simulink model "Autopilot"  (R2024a)
settings: Solver=ode4  StartTime=0.0  StopTime=1800  FixedStep=0.01  RelTol=1e-3
values from neighbouring files (symbols this model uses):
  A_lateral = [Yv, Yp+wo, Yr-u_0, g*cos(theta_0), 0 ... (first row only)    [main.m]
  A_longitudinal = [Xu, Xw,-w_0, -g*cos(theta_0) ... (first row only)    [main.m]
  B_lateral = [Yda, Ydr ... (first row only)    [main.m]
  B_longitudinal = [Xde, Xth ... (first row only)    [main.m]
  C_lateral = eye(5)    [main.m]
  C_longitudinal = eye(4)    [main.m]
  Control_Matrix = [0 Xde Xth 0 ... (first row only)    [main.m]
  D2R = pi/180    (= 0.0174532925199)    [main.m]
  D_lateral = zeros(5, 2)    [main.m]
  D_longitudinal = zeros(4, 2)    [main.m]
  g = aircraft_data(52)    [main.m]
  G = 1/(1-Ixz^2/(Ixx*Izz))    [LateralFunc.m]
  Ixx = aircraft_data(53)    [main.m]
  Iyy = aircraft_data(54)    [main.m]
  Izz = aircraft_data(55)    [main.m]
  m = aircraft_data(51)    [main.m]
  M_0 = [0;0;0]    [main.m]
  mg0 = m * g * [sin(s0(8)); -cos(s0(8)) * sin(s0(7)); -cos(s0(8)) * cos(s0(7))]    [main.m]
  p_0 = s0(4)    [main.m]
  phi_0 = s0(7)    [F_M_Calculation.m]    (also in main.m)
  psi_0 = s0(9)    [F_M_Calculation.m]    (also in main.m)
  q_0 = s0(5)    [main.m]
  R2D = 180/pi    (= 57.2957795131)    [main.m]
  r_0 = s0(6)    [main.m]
  s0 = aircraft_data(4:15)    [main.m]
  State_Matrix = [ Xu  0   Xw  0   0   0   0 ... (first row only)    [main.m]
  theta_0 = s0(8)    [F_M_Calculation.m]    (also in main.m)
  u_0 = s0(1)    [main.m]
  v_0 = s0(2)    [main.m]
  w_0 = s0(3)    [main.m]
  z_0 = s0(12)    [main.m]
undefined symbols (not defined in the file or in its folder): Earth, Receive, Send, so_struct, WGS84
libraries: cstblocks x20, simulink x3, aerolibfltsims x2, aerolibasang x2, aerolibtransform2 x1, SignalEditorBlockLib x1, shared6dof x1, dspsigops x1
settings Model: Creator=Abdelateef  LastModifiedBy=Abdelateef

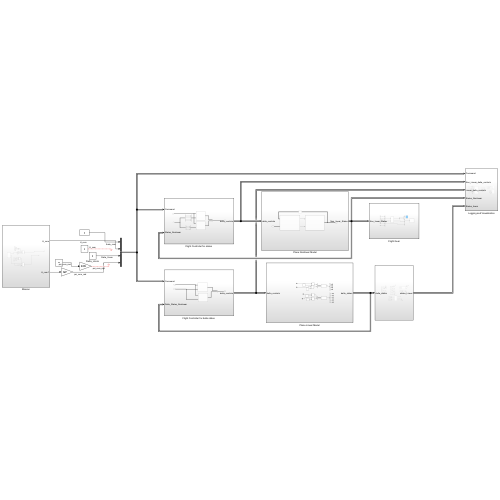
[thumbnail: Simulink's stored preview of the top-level diagram]
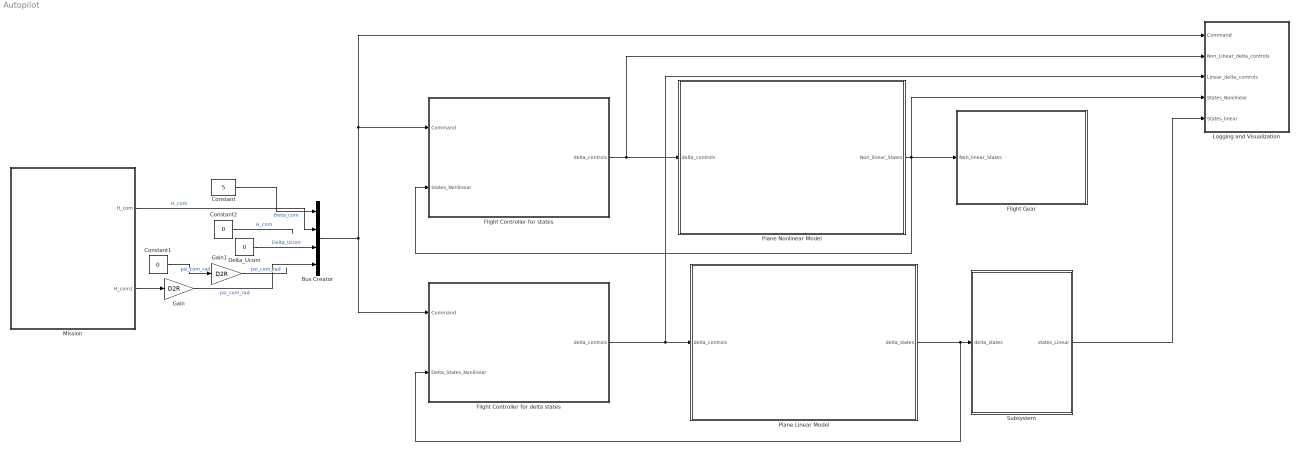
== system Autopilot ==
  Bus Creator : BusCreator  Inputs=4
  Constant : Constant  Value=5
  Constant1 : Constant  Value=0
  Constant2 : Constant  Value=0
  Delta_Ucom : Constant  Value=0
  "Flight Controller for delta states " : Subsystem
  "Flight Controller for states " : Subsystem
  Flight Gear : Subsystem
  Gain : Gain  Gain=D2R
  Gain1 : Gain  Gain=D2R
  Logging and Visualization : Subsystem
  Mission : Subsystem
  Plane Linear Model : Subsystem
  Plane Nonlinear Model : Subsystem
  Subsystem : Subsystem
  wires:
  "Flight Controller for states "/1(delta_controls) -> Logging and Visualization/2(Non_Linear_delta_controls), Plane Nonlinear Model/1(delta_controls)
  Plane Nonlinear Model/1(Non_linear_States) -> "Flight Controller for states "/2(States_Nonlinear), Flight Gear/1(Non_linear_States), Logging and Visualization/4(States_Nonlinear)
  Plane Linear Model/1(delta_states) -> "Flight Controller for delta states "/2(Delta_States_Nonlinear), Subsystem/1(delta_states)
  Bus Creator/1 -> Logging and Visualization/1(Command), "Flight Controller for states "/1(Command), "Flight Controller for delta states "/1(Command)
  "Flight Controller for delta states "/1(delta_controls) -> Logging and Visualization/3(Linear_delta_controls), Plane Linear Model/1(delta_controls)
  Gain/1 -> Bus Creator/4  "psi_com_rad"
  Delta_Ucom/1 -> Bus Creator/3  "Delta_Ucom"
  Subsystem/1(states_Linear) -> Logging and Visualization/5(States_linear)
  Constant1/1 -> Gain1/1  "psi_com_rad"
  Constant/1 -> Bus Creator/1  "theta_com"
  Gain1/1 -> ?  "psi_com_rad"
  Constant2/1 -> ?  "H_com"
  Mission/1(H_com) -> Bus Creator/2  "H_com"
  Mission/2(H_com1) -> Gain/1

== system Autopilot/Flight Controller for delta states  ==
  Command : Inport
  Delta_States_Nonlinear : Inport  Port=2
  Bus Creator : BusCreator  Inputs=2
  Lateral Controller : Subsystem
  Longitudinal Controller : Subsystem
  delta_controls : Outport
  wires:
  Lateral Controller/1(Latr_control_actions) -> Bus Creator/2  "Latr_control_actions"
  Longitudinal Controller/1(long_control_actions) -> Bus Creator/1  "long_control_actions"
  Bus Creator/1 -> delta_controls/1
  Command/1 -> Lateral Controller/1(Command), Longitudinal Controller/1(Command)
  Delta_States_Nonlinear/1 -> Lateral Controller/2(delta_states), Longitudinal Controller/2(delta_states)

== system Autopilot/Flight Controller for states  ==
  Command : Inport
  States_Nonlinear : Inport  Port=2
  Bus Creator : BusCreator  Inputs=5
  Bus Creator1 : BusCreator  Inputs=3
  Bus Creator2 : BusCreator  Inputs=2
  Bus Selector : BusSelector  OutputSignals=u,w,q,theta,H
  Bus Selector1 : BusSelector  OutputSignals=phi,psi,r
  Lateral Controller : Subsystem
  Longitudinal Controller : Subsystem
  delta_controls : Outport
  wires:
  Lateral Controller/1(Latr_control_actions) -> Bus Creator2/2  "Latr_control_actions"
  Longitudinal Controller/1(long_control_actions) -> Bus Creator2/1  "long_control_actions"
  Bus Creator2/1 -> delta_controls/1
  Command/1 -> Lateral Controller/1(Command), Longitudinal Controller/1(Command)
  States_Nonlinear/1 -> Bus Selector/1, Bus Selector1/1
  Bus Selector/1 -> Bus Creator/1  "<u>"
  Bus Selector/2 -> Bus Creator/2  "<w>"
  Bus Selector/3 -> Bus Creator/3  "<q>"
  Bus Selector/4 -> Bus Creator/4  "<theta>"
  Bus Selector/5 -> Bus Creator/5  "<H>"
  Bus Creator/1 -> Longitudinal Controller/2(States_long)
  Bus Selector1/3 -> Bus Creator1/3  "<r>"
  Bus Selector1/2 -> Bus Creator1/2  "<psi>"
  Bus Selector1/1 -> Bus Creator1/1  "<phi>"
  Bus Creator1/1 -> Lateral Controller/2(States_later)

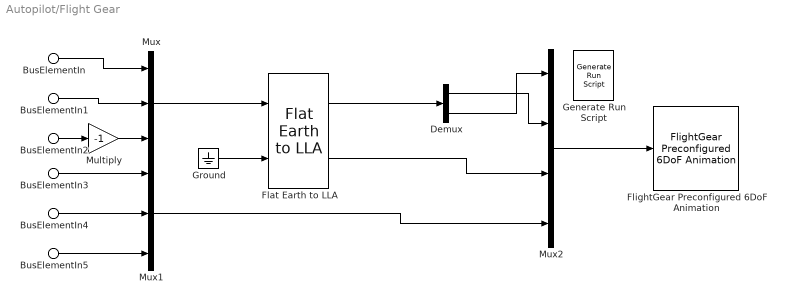
== system Autopilot/Flight Gear ==
  BusElementIn : Inport  PortName=Non_linear_States  Element=x
  BusElementIn1 : Inport  PortName=Non_linear_States  Element=y
  BusElementIn2 : Inport  PortName=Non_linear_States  Element=H
  BusElementIn3 : Inport  PortName=Non_linear_States  Element=phi
  BusElementIn4 : Inport  PortName=Non_linear_States  Element=theta
  BusElementIn5 : Inport  PortName=Non_linear_States  Element=psi
  Demux : Demux  Outputs=2
  Flat Earth to LLA : aerolibtransform2/Flat Earth to LLA  units=Metric (MKS)  ptype=Earth (WGS84)  F=1/298.257223563  R=6378137  refPosPort=off  LL0=[0 10]  psi=0
  FlightGear Preconfigured 6DoF Animation : aerolibfltsims/FlightGear Preconfigured 6DoF Animation  xFlightGearVersion=v2019.1  DestinationIpAddress=127.0.0.1  DestinationPort=5502  SampleTime=0.01  packetVersion=24
  Generate Run Script : aerolibfltsims/Generate Run Script  Architecture=Win64  dataFlow=Send-Receive  GeometryModelName=747-400  AirportId=LOWI  RunwayId=10L  InitialAltitude=-z_0  InitialHeading=psi_0  OffsetDistance=4.72  OffsetAzimuth=0  InstallScenery=off  DisableShaders=off  OriginAddress=127.0.0.1  DestinationPort=5502  OriginPort=5505  LocalAddress=127.0.0.1  OutputFileName=runfg.bat  FlightGearBaseDirectory=G:\FlightGear
  Ground : Ground
  Multiply : Gain  Gain=-1
  Mux : Mux  Inputs=3
  Mux1 : Mux  Inputs=3
  Mux2 : Mux
  wires:
  BusElementIn2/1 -> Multiply/1
  Multiply/1 -> Mux/3
  BusElementIn1/1 -> Mux/2
  BusElementIn/1 -> Mux/1
  Mux/1 -> Flat Earth to LLA/1
  Ground/1 -> Flat Earth to LLA/2
  BusElementIn3/1 -> Mux1/1
  BusElementIn4/1 -> Mux1/2
  BusElementIn5/1 -> Mux1/3
  Flat Earth to LLA/1 -> Demux/1
  Demux/2 -> Mux2/1
  Demux/1 -> Mux2/2
  Mux2/1 -> FlightGear Preconfigured 6DoF Animation/1
  Flat Earth to LLA/2 -> Mux2/3
  Mux1/1 -> Mux2/4

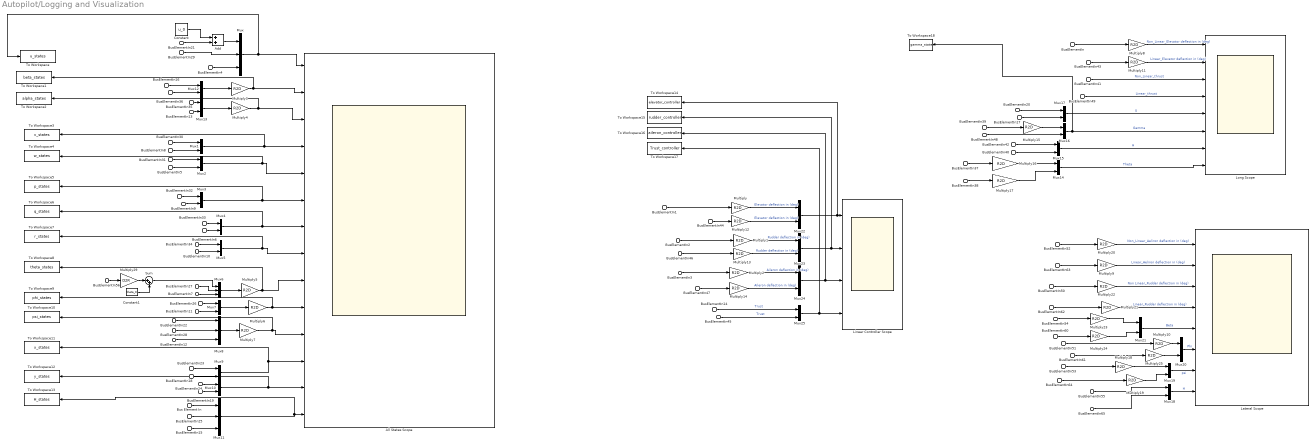
== system Autopilot/Logging and Visualization ==
  Bus Element In : Inport  PortName=Command  Element=H_com
  BusElementIn21 : Inport  PortName=Command  Element=Delta_Ucom
  BusElementIn22 : Inport  PortName=Command  Element=psi_com_rad
  BusElementIn56 : Inport  PortName=Command  Element=theta_com
  BusElementIn1 : Inport  Port=2  PortName=Non_Linear_delta_controls  Element=long_control_actions.delta_elevator(rad)
  BusElementIn : Inport  Port=2  PortName=Non_Linear_delta_controls  Element=long_control_actions.delta_elevator(rad)
  BusElementIn14 : Inport  Port=2  PortName=Non_Linear_delta_controls  Element=long_control_actions.delta_thrust
  BusElementIn41 : Inport  Port=2  PortName=Non_Linear_delta_controls  Element=long_control_actions.delta_thrust
  BusElementIn2 : Inport  Port=2  PortName=Non_Linear_delta_controls  Element=Latr_control_actions.delta_rudder(rad)
  BusElementIn50 : Inport  Port=2  PortName=Non_Linear_delta_controls  Element=Latr_control_actions.delta_rudder(rad)
  BusElementIn3 : Inport  Port=2  PortName=Non_Linear_delta_controls  Element=Latr_control_actions.delta_aileron(rad)
  BusElementIn52 : Inport  Port=2  PortName=Non_Linear_delta_controls  Element=Latr_control_actions.delta_aileron(rad)
  BusElementIn43 : Inport  Port=3  PortName=Linear_delta_controls  Element=long_control_actions.delta_elevator(rad)
  BusElementIn44 : Inport  Port=3  PortName=Linear_delta_controls  Element=long_control_actions.delta_elevator(rad)
  BusElementIn45 : Inport  Port=3  PortName=Linear_delta_controls  Element=long_control_actions.delta_thrust
  BusElementIn49 : Inport  Port=3  PortName=Linear_delta_controls  Element=long_control_actions.delta_thrust
  BusElementIn46 : Inport  Port=3  PortName=Linear_delta_controls  Element=Latr_control_actions.delta_rudder(rad)
  BusElementIn62 : Inport  Port=3  PortName=Linear_delta_controls  Element=Latr_control_actions.delta_rudder(rad)
  BusElementIn47 : Inport  Port=3  PortName=Linear_delta_controls  Element=Latr_control_actions.delta_aileron(rad)
  BusElementIn63 : Inport  Port=3  PortName=Linear_delta_controls  Element=Latr_control_actions.delta_aileron(rad)
  BusElementIn23 : Inport  Port=4  PortName=States_Nonlinear  Element=x
  BusElementIn24 : Inport  Port=4  PortName=States_Nonlinear  Element=y
  BusElementIn25 : Inport  Port=4  PortName=States_Nonlinear  Element=H
  BusElementIn42 : Inport  Port=4  PortName=States_Nonlinear  Element=H
  BusElementIn55 : Inport  Port=4  PortName=States_Nonlinear  Element=H
  BusElementIn26 : Inport  Port=4  PortName=States_Nonlinear  Element=phi
  BusElementIn51 : Inport  Port=4  PortName=States_Nonlinear  Element=phi
  BusElementIn27 : Inport  Port=4  PortName=States_Nonlinear  Element=theta
  BusElementIn37 : Inport  Port=4  PortName=States_Nonlinear  Element=theta
  BusElementIn28 : Inport  Port=4  PortName=States_Nonlinear  Element=psi
  BusElementIn53 : Inport  Port=4  PortName=States_Nonlinear  Element=psi
  BusElementIn29 : Inport  Port=4  PortName=States_Nonlinear  Element=u
  BusElementIn17 : Inport  Port=4  PortName=States_Nonlinear  Element=u
  BusElementIn30 : Inport  Port=4  PortName=States_Nonlinear  Element=v
  BusElementIn31 : Inport  Port=4  PortName=States_Nonlinear  Element=w
  BusElementIn32 : Inport  Port=4  PortName=States_Nonlinear  Element=p
  BusElementIn33 : Inport  Port=4  PortName=States_Nonlinear  Element=q
  BusElementIn34 : Inport  Port=4  PortName=States_Nonlinear  Element=r
  BusElementIn35 : Inport  Port=4  PortName=States_Nonlinear  Element=alpha
  BusElementIn36 : Inport  Port=4  PortName=States_Nonlinear  Element=Beta
  BusElementIn54 : Inport  Port=4  PortName=States_Nonlinear  Element=Beta
  BusElementIn39 : Inport  Port=4  PortName=States_Nonlinear  Element=gamma
  BusElementIn12 : Inport  Port=5  PortName=States_linear  Element=psi
  BusElementIn64 : Inport  Port=5  PortName=States_linear  Element=psi
  BusElementIn6 : Inport  Port=5  PortName=States_linear  Element=q
  BusElementIn4 : Inport  Port=5  PortName=States_linear  Element=u
  BusElementIn20 : Inport  Port=5  PortName=States_linear  Element=u
  BusElementIn5 : Inport  Port=5  PortName=States_linear  Element=w
  BusElementIn7 : Inport  Port=5  PortName=States_linear  Element=theta
  BusElementIn38 : Inport  Port=5  PortName=States_linear  Element=theta
  BusElementIn8 : Inport  Port=5  PortName=States_linear  Element=v
  BusElementIn9 : Inport  Port=5  PortName=States_linear  Element=p
  BusElementIn10 : Inport  Port=5  PortName=States_linear  Element=r
  BusElementIn11 : Inport  Port=5  PortName=States_linear  Element=phi
  BusElementIn61 : Inport  Port=5  PortName=States_linear  Element=phi
  BusElementIn13 : Inport  Port=5  PortName=States_linear  Element=alpha_(rad)
  BusElementIn15 : Inport  Port=5  PortName=States_linear  Element=H
  BusElementIn40 : Inport  Port=5  PortName=States_linear  Element=H
  BusElementIn65 : Inport  Port=5  PortName=States_linear  Element=H
  BusElementIn16 : Inport  Port=5  PortName=States_linear  Element=beta_(rad)
  BusElementIn60 : Inport  Port=5  PortName=States_linear  Element=beta_(rad)
  BusElementIn18 : Inport  Port=5  PortName=States_linear  Element=x
  BusElementIn19 : Inport  Port=5  PortName=States_linear  Element=y
  BusElementIn48 : Inport  Port=5  PortName=States_linear  Element=gamma_deg
  Add : Sum
  All States Scope : Scope  NumInputPorts=14
  Constant : Constant  Value=u_0
  Constant1 : Constant  Value=theta_0
  Lateral Scope : Scope  NumInputPorts=8
  Linear Controller Scope : Scope  NumInputPorts=4
  Long Scope : Scope  NumInputPorts=8
  Multiply{,1..25} (26 alike) : Gain  Gain=R2D
  Multiply29 : Gain  Gain=D2R
  Mux{,6,8,11} (4 alike) : Mux  Inputs=3
  Mux{1..5,7,9..10,12..25} (22 alike) : Mux  Inputs=2
  Sum : Sum  Inputs=|++
  To Workspace : ToWorkspace  VariableName=u_states  SaveFormat=Timeseries  SampleTime=-1
  To Workspace1 : ToWorkspace  VariableName=beta_states  SaveFormat=Timeseries  SampleTime=-1
  To Workspace10 : ToWorkspace  VariableName=psi_states  SaveFormat=Timeseries  SampleTime=-1
  To Workspace11 : ToWorkspace  VariableName=x_states  SaveFormat=Timeseries  SampleTime=-1
  To Workspace12 : ToWorkspace  VariableName=y_states  SaveFormat=Timeseries  SampleTime=-1
  To Workspace13 : ToWorkspace  VariableName=H_states  SaveFormat=Timeseries  SampleTime=-1
  To Workspace14 : ToWorkspace  VariableName=elevator_controller  SaveFormat=Timeseries  SampleTime=-1
  To Workspace15 : ToWorkspace  VariableName=rudder_controller  SaveFormat=Timeseries  SampleTime=-1
  To Workspace16 : ToWorkspace  VariableName=aileron_controller  SaveFormat=Timeseries  SampleTime=-1
  To Workspace17 : ToWorkspace  VariableName=Trust_controller  SaveFormat=Timeseries  SampleTime=-1
  To Workspace18 : ToWorkspace  VariableName=gamma_states  SaveFormat=Timeseries  SampleTime=-1
  To Workspace2 : ToWorkspace  VariableName=alpha_states  SaveFormat=Timeseries  SampleTime=-1
  To Workspace3 : ToWorkspace  VariableName=v_states  SaveFormat=Timeseries  SampleTime=-1
  To Workspace4 : ToWorkspace  VariableName=w_states  SaveFormat=Timeseries  SampleTime=-1
  To Workspace5 : ToWorkspace  VariableName=p_states  SaveFormat=Timeseries  SampleTime=-1
  To Workspace6 : ToWorkspace  VariableName=q_states  SaveFormat=Timeseries  SampleTime=-1
  To Workspace7 : ToWorkspace  VariableName=r_states  SaveFormat=Timeseries  SampleTime=-1
  To Workspace8 : ToWorkspace  VariableName=theta_states  SaveFormat=Timeseries  SampleTime=-1
  To Workspace9 : ToWorkspace  VariableName=phi_states  SaveFormat=Timeseries  SampleTime=-1
  wires:
  BusElementIn1/1 -> Multiply/1
  BusElementIn2/1 -> Multiply1/1
  BusElementIn3/1 -> Multiply2/1
  Multiply/1 -> Mux22/1  "Elevator deflection in (deg)"
  Multiply1/1 -> Mux23/1  "Rudder deflection in (deg)"
  Multiply2/1 -> Mux24/1  "Aileron deflection in (deg)"
  Constant/1 -> Add/1
  BusElementIn21/1 -> Add/2
  Add/1 -> Mux/1
  BusElementIn4/1 -> Mux/3
  BusElementIn29/1 -> Mux/2
  BusElementIn8/1 -> Mux1/2
  BusElementIn30/1 -> Mux1/1
  BusElementIn5/1 -> Mux2/2
  BusElementIn31/1 -> Mux2/1
  BusElementIn9/1 -> Mux3/2
  BusElementIn32/1 -> Mux3/1
  BusElementIn6/1 -> Mux4/2
  BusElementIn33/1 -> Mux4/1
  BusElementIn34/1 -> Mux5/1
  BusElementIn10/1 -> Mux5/2
  BusElementIn7/1 -> Mux6/3
  BusElementIn27/1 -> Mux6/2
  BusElementIn11/1 -> Mux7/2
  BusElementIn26/1 -> Mux7/1
  BusElementIn12/1 -> Mux8/3
  BusElementIn28/1 -> Mux8/2
  BusElementIn22/1 -> Mux8/1
  BusElementIn18/1 -> Mux9/2
  BusElementIn23/1 -> Mux9/1
  BusElementIn24/1 -> Mux10/1
  BusElementIn19/1 -> Mux10/2
  BusElementIn15/1 -> Mux11/3
  Bus Element In/1 -> Mux11/1
  BusElementIn16/1 -> Mux12/1
  BusElementIn36/1 -> Mux12/2
  BusElementIn35/1 -> Mux13/1
  BusElementIn13/1 -> Mux13/2
  Mux/1 -> All States Scope/1, To Workspace/1
  Mux12/1 -> Multiply3/1
  Mux13/1 -> Multiply4/1
  Mux6/1 -> Multiply5/1
  Mux7/1 -> Multiply6/1
  Mux8/1 -> Multiply7/1
  BusElementIn14/1 -> Mux25/1  "Trust"
  Multiply8/1 -> Long Scope/1  "Non_Linear_Elevator deflection in (deg)"
  BusElementIn/1 -> Multiply8/1
  BusElementIn38/1 -> Multiply17/1
  BusElementIn37/1 -> Multiply16/1
  Mux16/1 -> Long Scope/6, To Workspace18/1  "Gamma"
  Mux15/1 -> Long Scope/7  "H"
  BusElementIn40/1 -> Mux15/2
  BusElementIn42/1 -> Mux15/1
  BusElementIn48/1 -> Mux16/2
  Mux17/1 -> Long Scope/5  "U"
  BusElementIn17/1 -> Mux17/2
  BusElementIn20/1 -> Mux17/1
  BusElementIn43/1 -> Multiply11/1
  Multiply11/1 -> Long Scope/2  "Linear_Elevator deflection in (deg)"
  Multiply13/1 -> Mux23/2  "Rudder deflection in (deg)"
  Multiply14/1 -> Mux24/2  "Aileron deflection in (deg)"
  BusElementIn45/1 -> Mux25/2  "Trust"
  Multiply12/1 -> Mux22/2  "Elevator deflection in (deg)"
  BusElementIn44/1 -> Multiply12/1
  BusElementIn46/1 -> Multiply13/1
  BusElementIn47/1 -> Multiply14/1
  BusElementIn39/1 -> Multiply15/1
  Multiply15/1 -> Mux16/1
  Multiply16/1 -> Mux14/1
  Multiply17/1 -> Mux14/2
  Mux14/1 -> Long Scope/8  "Theta"
  BusElementIn41/1 -> Long Scope/3  "Non_Linear_thrust"
  BusElementIn49/1 -> Long Scope/4  "Linear_thrust"
  BusElementIn55/1 -> Mux18/1
  Mux18/1 -> Lateral Scope/8  "H"
  Mux21/1 -> Lateral Scope/5  "Beta"
  Multiply9/1 -> Lateral Scope/2  "Linear_Aeliron deflection in (deg)"
  Mux19/1 -> Lateral Scope/7  "psi"
  Multiply20/1 -> Lateral Scope/1  "Non_Linear_Aeliron deflection in (deg)"
  Mux20/1 -> Lateral Scope/6  "Phi"
  Multiply10/1 -> Mux20/1
  BusElementIn63/1 -> Multiply9/1
  BusElementIn50/1 -> Multiply22/1
  BusElementIn62/1 -> Multiply21/1
  Multiply21/1 -> Lateral Scope/4  "Linear_Rudder deflection in (deg)"
  BusElementIn52/1 -> Multiply20/1
  Multiply22/1 -> Lateral Scope/3  "Non Linear_Rudder deflection in (deg)"
  Multiply23/1 -> Mux21/1
  Multiply24/1 -> Mux21/2
  Multiply25/1 -> Mux20/2
  Multiply18/1 -> Mux19/1
  Multiply19/1 -> Mux19/2
  BusElementIn54/1 -> Multiply23/1
  BusElementIn51/1 -> Multiply10/1
  BusElementIn53/1 -> Multiply18/1
  BusElementIn60/1 -> Multiply24/1
  BusElementIn61/1 -> Multiply25/1
  BusElementIn64/1 -> Multiply19/1
  BusElementIn65/1 -> Mux18/2
  Multiply3/1 -> All States Scope/2, To Workspace1/1
  Multiply4/1 -> To Workspace2/1, All States Scope/3
  Mux1/1 -> To Workspace3/1, All States Scope/4
  Mux2/1 -> To Workspace4/1, All States Scope/5
  Mux3/1 -> To Workspace5/1, All States Scope/6
  Mux4/1 -> To Workspace6/1, All States Scope/7
  Mux5/1 -> To Workspace7/1, All States Scope/8
  Multiply5/1 -> To Workspace8/1, All States Scope/9
  Multiply6/1 -> To Workspace9/1, All States Scope/10
  Multiply7/1 -> To Workspace10/1, All States Scope/11
  Mux9/1 -> All States Scope/12, To Workspace11/1
  Mux10/1 -> To Workspace12/1, All States Scope/13
  Mux22/1 -> To Workspace14/1, Linear Controller Scope/1
  Mux23/1 -> To Workspace15/1, Linear Controller Scope/2
  Mux24/1 -> To Workspace16/1, Linear Controller Scope/3
  Mux25/1 -> To Workspace17/1, Linear Controller Scope/4
  BusElementIn56/1 -> Multiply29/1
  Mux11/1 -> To Workspace13/1, All States Scope/14
  BusElementIn25/1 -> Mux11/2
  Multiply29/1 -> Sum/1
  Sum/1 -> Mux6/1
  Constant1/1 -> Sum/2

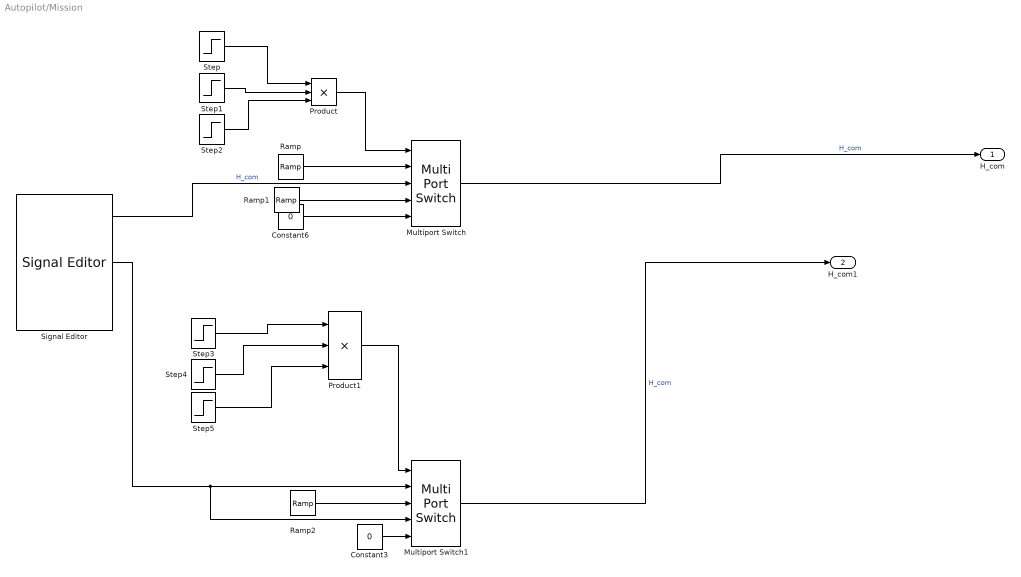
== system Autopilot/Mission ==
  Constant3 : Constant  Value=0
  Constant6 : Constant  Value=0
  Multiport Switch : MultiPortSwitch  Inputs=4  SaturateOnIntegerOverflow=off  InputSameDT=off
  Multiport Switch1 : MultiPortSwitch  Inputs=4  SaturateOnIntegerOverflow=off  InputSameDT=off
  Product : Product  Inputs=3
  Product1 : Product  Inputs=3
  Ramp : simulink/Sources/Ramp  slope=25  start=0  InitialOutput=0
  Ramp1 : simulink/Sources/Ramp  slope=-25.25  start=1000  InitialOutput=10100
  Ramp2 : simulink/Sources/Ramp  slope=3/2  start=520  InitialOutput=0
  Signal Editor : SignalEditorBlockLib/Signal Editor  FileName=F:\University of Science and Technology at Zewail City\SPC\Level4\Autopilot\Task7\Mission_input.mat  ActiveScenario=Scenario  ActiveSignal=H_com  IsBus=off  OutputBusObjectStr=Bus: BusObject  SampleTime=0  Interpolate=off  ZeroCross=off  OutputAfterFinalValue=Setting to zero  Unit=inherit  PreserveSignalName=on  ApplySigPropsToAllScenarios=off  ApplySigPropsToAllSignals=on
  Step : Step  Time=400  Before=1  After=2  SampleTime=0
  Step1 : Step  Time=1000.  Before=1  After=1.5  SampleTime=0
  Step2 : Step  Time=1400  Before=1  After=4/3  SampleTime=0
  Step3 : Step  Time=520  Before=1  After=2  SampleTime=0
  Step4 : Step  Time=760  Before=1  After=1.5  SampleTime=0
  Step5 : Step  Time=1400  Before=1  After=4/3  SampleTime=0
  H_com : Outport
  H_com1 : Outport  Port=2
  wires:
  Signal Editor/2 -> Multiport Switch1/4, Multiport Switch1/2
  Constant6/1 -> Multiport Switch/5
  Ramp/1 -> Multiport Switch/2
  Product/1 -> Multiport Switch/1
  Step1/1 -> Product/2
  Ramp1/1 -> Multiport Switch/4
  Multiport Switch/1 -> H_com/1  "H_com"
  Constant3/1 -> Multiport Switch1/5
  Multiport Switch1/1 -> H_com1/1  "H_com"
  Step/1 -> Product/1
  Signal Editor/1 -> Multiport Switch/3  "H_com"
  Step2/1 -> Product/3
  Product1/1 -> Multiport Switch1/1
  Step3/1 -> Product1/1
  Step4/1 -> Product1/2
  Step5/1 -> Product1/3
  Ramp2/1 -> Multiport Switch1/3

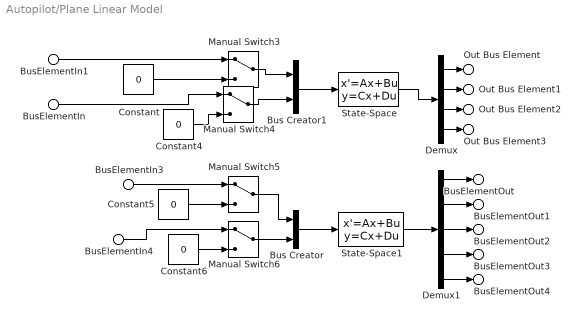
== system Autopilot/Plane Linear Model ==
  BusElementIn : Inport  PortName=delta_controls  Element=long_control_actions.delta_thrust
  BusElementIn1 : Inport  PortName=delta_controls  Element=long_control_actions.delta_elevator(rad)
  BusElementIn3 : Inport  PortName=delta_controls  Element=Latr_control_actions.delta_aileron(rad)
  BusElementIn4 : Inport  PortName=delta_controls  Element=Latr_control_actions.delta_rudder(rad)
  Bus Creator : BusCreator  Inputs=2
  Bus Creator1 : BusCreator  Inputs=2
  Constant{,4..6} (4 alike) : Constant  Value=0
  Demux : Demux
  Demux1 : Demux  Outputs=5
  Manual Switch{3..6} (4 alike) : ManualSwitch
  State-Space : StateSpace  A=A_longitudinal  B=B_longitudinal  C=C_longitudinal  D=D_longitudinal  InitialCondition=0  ParameterTunability=Unconstrained
  State-Space1 : StateSpace  A=A_lateral  B=B_lateral  C=C_lateral  D=D_lateral  InitialCondition=0  ParameterTunability=Unconstrained
  Out Bus Element : Outport  PortName=delta_states  Element=delta_u
  Out Bus Element1 : Outport  PortName=delta_states  Element=delta_w
  Out Bus Element2 : Outport  PortName=delta_states  Element=delta_q
  Out Bus Element3 : Outport  PortName=delta_states  Element=delta_theta(rad)
  BusElementOut : Outport  PortName=delta_states  Element=delta_v
  BusElementOut1 : Outport  PortName=delta_states  Element=delta_p
  BusElementOut2 : Outport  PortName=delta_states  Element=delta_r
  BusElementOut3 : Outport  PortName=delta_states  Element=delta_phi(rad)
  BusElementOut4 : Outport  PortName=delta_states  Element=delta_psi(rad)
  wires:
  Demux/3 -> Out Bus Element2/1
  State-Space/1 -> Demux/1
  Demux/4 -> Out Bus Element3/1
  Demux/2 -> Out Bus Element1/1
  Demux/1 -> Out Bus Element/1
  State-Space1/1 -> Demux1/1
  BusElementIn4/1 -> Manual Switch6/1
  Demux1/2 -> BusElementOut1/1
  Demux1/1 -> BusElementOut/1
  Demux1/4 -> BusElementOut3/1
  Bus Creator/1 -> State-Space1/1
  Demux1/5 -> BusElementOut4/1
  Demux1/3 -> BusElementOut2/1
  BusElementIn3/1 -> Manual Switch5/1
  BusElementIn/1 -> Manual Switch4/1
  BusElementIn1/1 -> Manual Switch3/1
  Bus Creator1/1 -> State-Space/1
  Constant4/1 -> Manual Switch4/2
  Manual Switch4/1 -> Bus Creator1/2
  Constant/1 -> Manual Switch3/2
  Manual Switch3/1 -> Bus Creator1/1
  Constant6/1 -> Manual Switch6/2
  Manual Switch6/1 -> Bus Creator/2
  Constant5/1 -> Manual Switch5/2
  Manual Switch5/1 -> Bus Creator/1

== system Autopilot/Plane Nonlinear Model ==
  delta_controls : Inport
  Aircraft Model : Subsystem
  Nonlinear RBD : Subsystem
  Unit Delay : UnitDelay  Commented=through  InitialCondition=so_struct  SampleTime=-1  HasFrameUpgradeWarning=on
  Non_linear_States : Outport
  wires:
  Aircraft Model/1(delta_forces) -> Nonlinear RBD/1(delta_forces)
  Aircraft Model/2(selta_Moments) -> Nonlinear RBD/2(delta_Moments)
  Nonlinear RBD/1(States) -> Non_linear_States/1, Unit Delay/1
  delta_controls/1 -> Aircraft Model/2(delta_controls)
  Unit Delay/1 -> Aircraft Model/1(State)

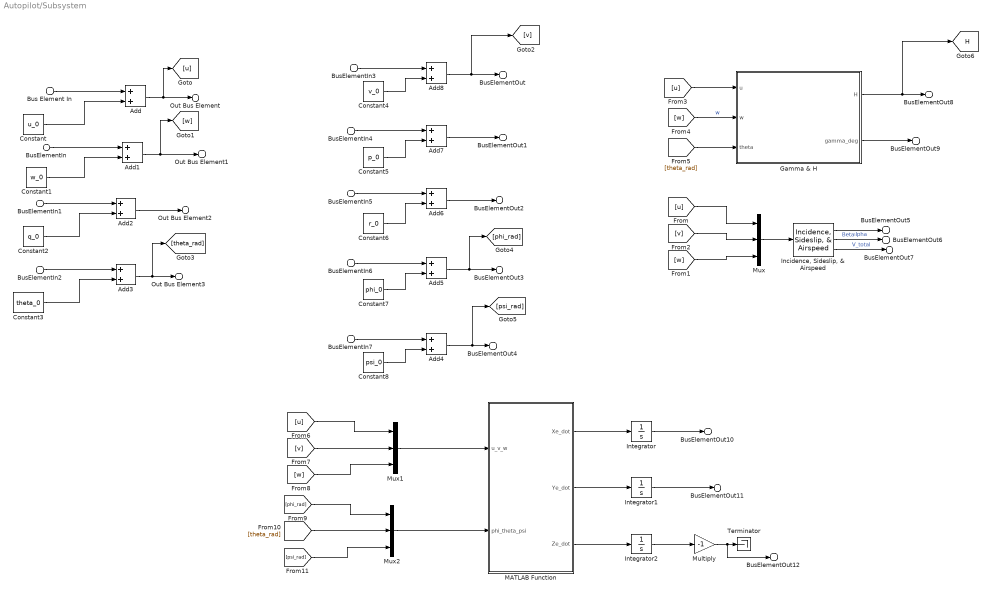
== system Autopilot/Subsystem ==
  Bus Element In : Inport  PortName=delta_states  Element=delta_u
  BusElementIn : Inport  PortName=delta_states  Element=delta_w
  BusElementIn1 : Inport  PortName=delta_states  Element=delta_q
  BusElementIn2 : Inport  PortName=delta_states  Element=delta_theta(rad)
  BusElementIn3 : Inport  PortName=delta_states  Element=delta_v
  BusElementIn4 : Inport  PortName=delta_states  Element=delta_p
  BusElementIn5 : Inport  PortName=delta_states  Element=delta_r
  BusElementIn6 : Inport  PortName=delta_states  Element=delta_phi(rad)
  BusElementIn7 : Inport  PortName=delta_states  Element=delta_psi(rad)
  Add{,1..8} (9 alike) : Sum
  Constant : Constant  Value=u_0
  Constant1 : Constant  Value=w_0
  Constant2 : Constant  Value=q_0
  Constant3 : Constant  Value=theta_0
  Constant4 : Constant  Value=v_0
  Constant5 : Constant  Value=p_0
  Constant6 : Constant  Value=r_0
  Constant7 : Constant  Value=phi_0
  Constant8 : Constant  Value=psi_0
  Gamma & H : Subsystem
  "Incidence, Sideslip, & Airspeed" : aerolibasang/Incidence, Sideslip, & Airspeed
  Integrator : Integrator
  Integrator1 : Integrator
  Integrator2 : Integrator
  MATLAB Function : MATLAB Function  TreatAsAtomicUnit=on
  Multiply : Gain  Gain=-1
  Mux : Mux  Inputs=3
  Mux1 : Mux  Inputs=3
  Mux2 : Mux  Inputs=3
  Terminator : Terminator
  Out Bus Element : Outport  PortName=states_Linear  Element=u
  Out Bus Element1 : Outport  PortName=states_Linear  Element=w
  Out Bus Element2 : Outport  PortName=states_Linear  Element=q
  Out Bus Element3 : Outport  PortName=states_Linear  Element=theta
  BusElementOut : Outport  PortName=states_Linear  Element=v
  BusElementOut1 : Outport  PortName=states_Linear  Element=p
  BusElementOut2 : Outport  PortName=states_Linear  Element=r
  BusElementOut3 : Outport  PortName=states_Linear  Element=phi
  BusElementOut4 : Outport  PortName=states_Linear  Element=psi
  BusElementOut5 : Outport  PortName=states_Linear  Element=alpha_(rad)
  BusElementOut6 : Outport  PortName=states_Linear  Element=beta_(rad)
  BusElementOut7 : Outport  PortName=states_Linear  Element=v_total
  BusElementOut8 : Outport  PortName=states_Linear  Element=H
  BusElementOut9 : Outport  PortName=states_Linear  Element=gamma_deg
  BusElementOut10 : Outport  PortName=states_Linear  Element=x
  BusElementOut11 : Outport  PortName=states_Linear  Element=y
  BusElementOut12 : Outport  PortName=states_Linear  Element=H2
  tag scope: H=global
  wires:
  Bus Element In/1 -> Add/1
  BusElementIn/1 -> Add1/1
  BusElementIn1/1 -> Add2/1
  BusElementIn2/1 -> Add3/1
  BusElementIn7/1 -> Add4/1
  BusElementIn6/1 -> Add5/1
  BusElementIn5/1 -> Add6/1
  BusElementIn4/1 -> Add7/1
  BusElementIn3/1 -> Add8/1
  Constant/1 -> Add/2
  Constant1/1 -> Add1/2
  Constant2/1 -> Add2/2
  Constant3/1 -> Add3/2
  Constant4/1 -> Add8/2
  Constant5/1 -> Add7/2
  Constant6/1 -> Add6/2
  Constant7/1 -> Add5/2
  Constant8/1 -> Add4/2
  Add5/1 -> [phi_rad], BusElementOut3/1
  Add7/1 -> BusElementOut1/1
  Add/1 -> [u], Out Bus Element/1
  Add6/1 -> BusElementOut2/1
  Add1/1 -> [w], Out Bus Element1/1
  Add2/1 -> Out Bus Element2/1
  Add3/1 -> [theta_rad], Out Bus Element3/1
  Add8/1 -> [v], BusElementOut/1
  Add4/1 -> [psi_rad], BusElementOut4/1
  Mux/1 -> "Incidence, Sideslip, & Airspeed"/1
  [v] -> Mux/2
  [u] -> Mux/1
  [w] -> Mux/3
  "Incidence, Sideslip, & Airspeed"/1 -> BusElementOut5/1  "alpha"
  "Incidence, Sideslip, & Airspeed"/3 -> BusElementOut7/1  "V_total"
  "Incidence, Sideslip, & Airspeed"/2 -> BusElementOut6/1  "Beta"
  [w] -> Gamma & H/2(w)  "w"
  Gamma & H/1(H) -> [H], BusElementOut8/1
  [theta_rad] -> Gamma & H/3(theta)
  [u] -> Gamma & H/1(u)
  Gamma & H/2(gamma_deg) -> BusElementOut9/1
  Mux1/1 -> MATLAB Function/1(u_v_w)
  [u] -> Mux1/1
  [v] -> Mux1/2
  [w] -> Mux1/3
  [psi_rad] -> Mux2/3
  [theta_rad] -> Mux2/2
  Mux2/1 -> MATLAB Function/2(phi_theta_psi)
  [phi_rad] -> Mux2/1
  MATLAB Function/1(Xe_dot) -> Integrator/1
  MATLAB Function/2(Ye_dot) -> Integrator1/1
  MATLAB Function/3(Ze_dot) -> Integrator2/1
  Integrator/1 -> BusElementOut10/1
  Integrator2/1 -> Multiply/1
  Integrator1/1 -> BusElementOut11/1
  Multiply/1 -> BusElementOut12/1, Terminator/1

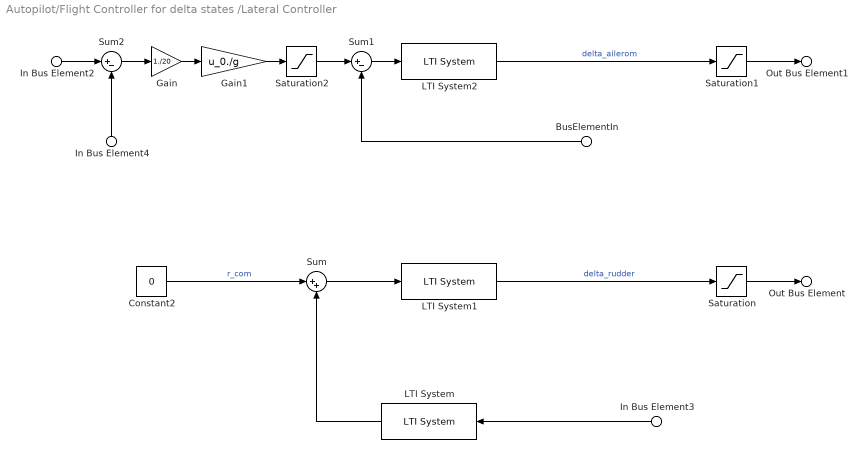
== system Autopilot/Flight Controller for delta states /Lateral Controller ==
  In Bus Element2 : Inport  PortName=Command  Element=psi_com_rad
  In Bus Element3 : Inport  Port=2  PortName=delta_states  Element=delta_r
  In Bus Element4 : Inport  Port=2  PortName=delta_states  Element=delta_psi(rad)
  BusElementIn : Inport  Port=2  PortName=delta_states  Element=delta_phi(rad)
  Constant2 : Constant  Value=0
  Gain : Gain  Gain=1./20
  Gain1 : Gain  Gain=u_0./g
  LTI System : cstblocks/LTI System  sys=HPF_YawDamper  IC=[]  PadeOrder=0
  LTI System1 : cstblocks/LTI System  sys=servo  IC=[]  PadeOrder=0
  LTI System2 : cstblocks/LTI System  sys=servo  IC=[]  PadeOrder=0
  Saturation : Saturate  UpperLimit=15*pi/180  LowerLimit=-15*pi/180
  Saturation1 : Saturate  UpperLimit=50*pi/180  LowerLimit=-50*pi/180
  Saturation2 : Saturate  UpperLimit=30*pi/180  LowerLimit=-30*pi/180
  Sum : Sum  Inputs=|++
  Sum1 : Sum  Inputs=|+-
  Sum2 : Sum  Inputs=|+-
  Out Bus Element : Outport  PortName=Latr_control_actions  Element=delta_rudder(rad)
  Out Bus Element1 : Outport  PortName=Latr_control_actions  Element=delta_aileron(rad)
  wires:
  BusElementIn/1 -> Sum1/2
  Constant2/1 -> Sum/1  "r_com"
  In Bus Element3/1 -> LTI System/1
  In Bus Element2/1 -> Sum2/1
  Saturation2/1 -> Sum1/1
  LTI System2/1 -> Saturation1/1  "delta_ailerom"
  Saturation1/1 -> Out Bus Element1/1
  Sum/1 -> LTI System1/1
  Sum2/1 -> Gain/1
  Sum1/1 -> LTI System2/1
  LTI System1/1 -> Saturation/1  "delta_rudder"
  In Bus Element4/1 -> Sum2/2
  Gain1/1 -> Saturation2/1
  Saturation/1 -> Out Bus Element/1
  LTI System/1 -> Sum/2
  Gain/1 -> Gain1/1

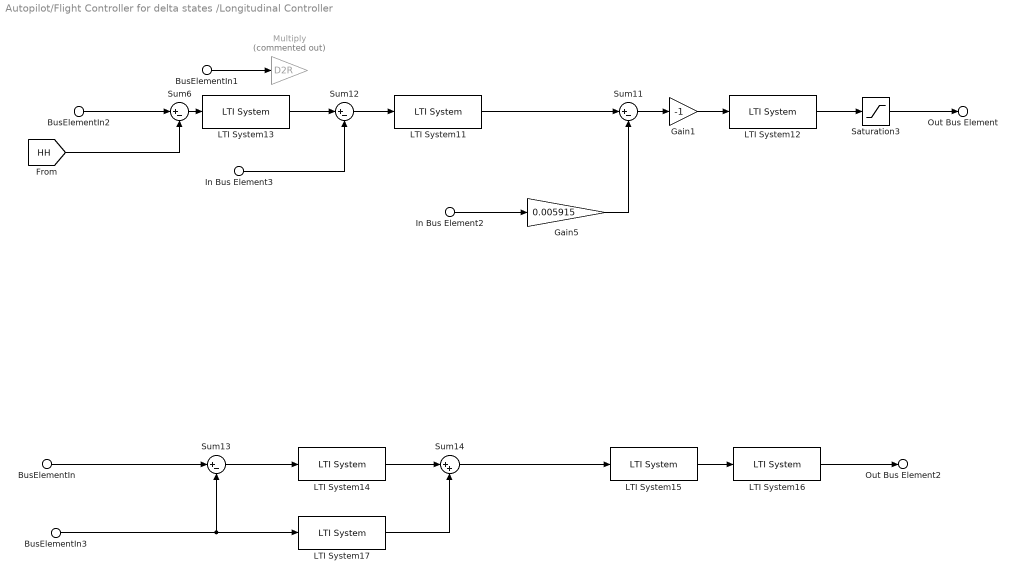
== system Autopilot/Flight Controller for delta states /Longitudinal Controller ==
  BusElementIn : Inport  PortName=Command  Element=Delta_Ucom
  BusElementIn2 : Inport  PortName=Command  Element=H_com
  BusElementIn1 : Inport  PortName=Command  Element=theta_com
  In Bus Element2 : Inport  Port=2  PortName=delta_states  Element=delta_q
  In Bus Element3 : Inport  Port=2  PortName=delta_states  Element=delta_theta(rad)
  BusElementIn3 : Inport  Port=2  PortName=delta_states  Element=delta_u
  Gain1 : Gain  Gain=-1
  Gain5 : Gain  Gain=0.005915
  LTI System11 : cstblocks/LTI System  sys=PI_Pitch  IC=[]  PadeOrder=0
  LTI System12 : cstblocks/LTI System  sys=servo  IC=[]  PadeOrder=0
  LTI System13 : cstblocks/LTI System  sys=PI_altitude  IC=[]  PadeOrder=0
  LTI System14 : cstblocks/LTI System  sys=C1  IC=[]  PadeOrder=0
  LTI System15 : cstblocks/LTI System  sys=servo  IC=[]  PadeOrder=0
  LTI System16 : cstblocks/LTI System  sys=engine_timelag  IC=[]  PadeOrder=0
  LTI System17 : cstblocks/LTI System  sys=C2  IC=[]  PadeOrder=0
  Multiply : Gain  Commented=on  Gain=D2R
  Saturation3 : Saturate  UpperLimit=25*pi/180  LowerLimit=-25*pi/180
  Sum{6,11..13} (4 alike) : Sum  Inputs=|+-
  Sum14 : Sum  Inputs=|++
  Out Bus Element : Outport  PortName=long_control_actions  Element=delta_elevator(rad)
  Out Bus Element2 : Outport  PortName=long_control_actions  Element=delta_thrust
  wires:
  In Bus Element2/1 -> Gain5/1
  BusElementIn2/1 -> Sum6/1
  [HH] -> Sum6/2
  In Bus Element3/1 -> Sum12/2
  Gain1/1 -> LTI System12/1
  Sum11/1 -> Gain1/1
  Sum12/1 -> LTI System11/1
  Sum6/1 -> LTI System13/1
  LTI System11/1 -> Sum11/1
  BusElementIn3/1 -> Sum13/2, LTI System17/1
  LTI System17/1 -> Sum14/2
  Sum13/1 -> LTI System14/1
  Gain5/1 -> Sum11/2
  Sum14/1 -> LTI System15/1
  LTI System14/1 -> Sum14/1
  LTI System15/1 -> LTI System16/1
  LTI System12/1 -> Saturation3/1
  LTI System16/1 -> Out Bus Element2/1
  Saturation3/1 -> Out Bus Element/1
  BusElementIn/1 -> Sum13/1
  BusElementIn1/1 -> Multiply/1
  LTI System13/1 -> Sum12/1

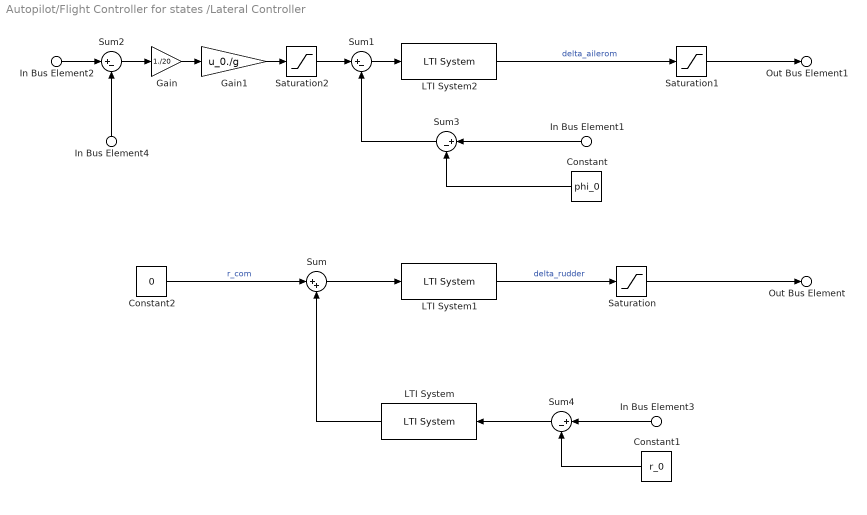
== system Autopilot/Flight Controller for states /Lateral Controller ==
  In Bus Element2 : Inport  PortName=Command  Element=psi_com_rad
  In Bus Element3 : Inport  Port=2  PortName=States_later  Element=r
  In Bus Element1 : Inport  Port=2  PortName=States_later  Element=phi
  In Bus Element4 : Inport  Port=2  PortName=States_later  Element=psi
  Constant : Constant  Value=phi_0
  Constant1 : Constant  Value=r_0
  Constant2 : Constant  Value=0
  Gain : Gain  Gain=1./20
  Gain1 : Gain  Gain=u_0./g
  LTI System : cstblocks/LTI System  sys=HPF_YawDamper  IC=[]  PadeOrder=0
  LTI System1 : cstblocks/LTI System  sys=servo  IC=[]  PadeOrder=0
  LTI System2 : cstblocks/LTI System  sys=servo  IC=[]  PadeOrder=0
  Saturation : Saturate  UpperLimit=15*pi/180  LowerLimit=-15*pi/180
  Saturation1 : Saturate  UpperLimit=50*pi/180  LowerLimit=-50*pi/180
  Saturation2 : Saturate  UpperLimit=30*pi/180  LowerLimit=-30*pi/180
  Sum : Sum  Inputs=|++
  Sum{1..4} (4 alike) : Sum  Inputs=|+-
  Out Bus Element : Outport  PortName=Latr_control_actions  Element=delta_rudder(rad)
  Out Bus Element1 : Outport  PortName=Latr_control_actions  Element=delta_aileron(rad)
  wires:
  Saturation2/1 -> Sum1/1
  Gain1/1 -> Saturation2/1
  In Bus Element2/1 -> Sum2/1
  LTI System1/1 -> Saturation/1  "delta_rudder"
  Gain/1 -> Gain1/1
  Sum1/1 -> LTI System2/1
  Sum/1 -> LTI System1/1
  LTI System/1 -> Sum/2
  In Bus Element4/1 -> Sum2/2
  Sum2/1 -> Gain/1
  In Bus Element1/1 -> Sum3/1
  LTI System2/1 -> Saturation1/1  "delta_ailerom"
  Sum3/1 -> Sum1/2
  Constant/1 -> Sum3/2
  Sum4/1 -> LTI System/1
  In Bus Element3/1 -> Sum4/1
  Constant1/1 -> Sum4/2
  Constant2/1 -> Sum/1  "r_com"
  Saturation/1 -> Out Bus Element/1
  Saturation1/1 -> Out Bus Element1/1

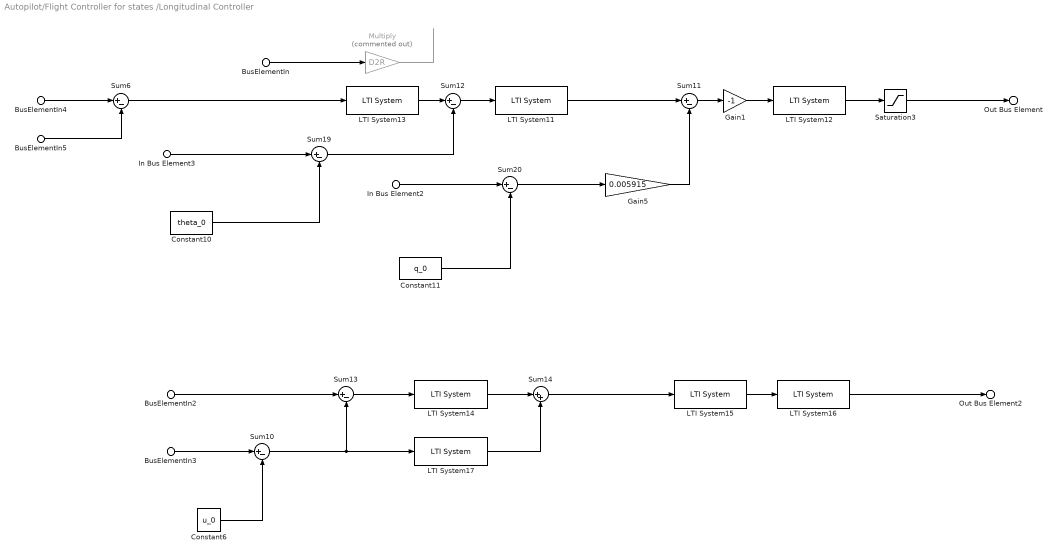
== system Autopilot/Flight Controller for states /Longitudinal Controller ==
  BusElementIn2 : Inport  PortName=Command  Element=Delta_Ucom
  BusElementIn4 : Inport  PortName=Command  Element=H_com
  BusElementIn : Inport  PortName=Command  Element=theta_com
  In Bus Element2 : Inport  Port=2  PortName=States_long  Element=q
  In Bus Element3 : Inport  Port=2  PortName=States_long  Element=theta
  BusElementIn3 : Inport  Port=2  PortName=States_long  Element=u
  BusElementIn5 : Inport  Port=2  PortName=States_long  Element=H
  Constant10 : Constant  Value=theta_0
  Constant11 : Constant  Value=q_0
  Constant6 : Constant  Value=u_0
  Gain1 : Gain  Gain=-1
  Gain5 : Gain  Gain=0.005915
  LTI System11 : cstblocks/LTI System  sys=PI_Pitch  IC=[]  PadeOrder=0
  LTI System12 : cstblocks/LTI System  sys=servo  IC=[]  PadeOrder=0
  LTI System13 : cstblocks/LTI System  sys=PI_altitude  IC=[]  PadeOrder=0
  LTI System14 : cstblocks/LTI System  sys=C1  IC=[]  PadeOrder=0
  LTI System15 : cstblocks/LTI System  sys=servo  IC=[]  PadeOrder=0
  LTI System16 : cstblocks/LTI System  sys=engine_timelag  IC=[]  PadeOrder=0
  LTI System17 : cstblocks/LTI System  sys=C2  IC=[]  PadeOrder=0
  Multiply : Gain  Commented=on  Gain=D2R
  Saturation3 : Saturate  UpperLimit=25*pi/180  LowerLimit=-25*pi/180
  Sum{6,10..13,19..20} (7 alike) : Sum  Inputs=|+-
  Sum14 : Sum  Inputs=|++
  Out Bus Element : Outport  PortName=long_control_actions  Element=delta_elevator(rad)
  Out Bus Element2 : Outport  PortName=long_control_actions  Element=delta_thrust
  wires:
  BusElementIn2/1 -> Sum13/1
  In Bus Element3/1 -> Sum19/1
  In Bus Element2/1 -> Sum20/1
  BusElementIn3/1 -> Sum10/1
  Constant6/1 -> Sum10/2
  BusElementIn4/1 -> Sum6/1
  BusElementIn5/1 -> Sum6/2
  Sum12/1 -> LTI System11/1
  Sum11/1 -> Gain1/1
  Constant10/1 -> Sum19/2
  Constant11/1 -> Sum20/2
  Sum19/1 -> Sum12/2
  LTI System11/1 -> Sum11/1
  LTI System12/1 -> Saturation3/1
  Sum20/1 -> Gain5/1
  Gain1/1 -> LTI System12/1
  Gain5/1 -> Sum11/2
  Sum13/1 -> LTI System14/1
  LTI System16/1 -> Out Bus Element2/1
  Sum14/1 -> LTI System15/1
  LTI System14/1 -> Sum14/1
  LTI System17/1 -> Sum14/2
  LTI System15/1 -> LTI System16/1
  Sum10/1 -> Sum13/2, LTI System17/1
  Sum6/1 -> LTI System13/1
  Saturation3/1 -> Out Bus Element/1
  BusElementIn/1 -> Multiply/1
  Multiply/1 -> ?
  LTI System13/1 -> Sum12/1

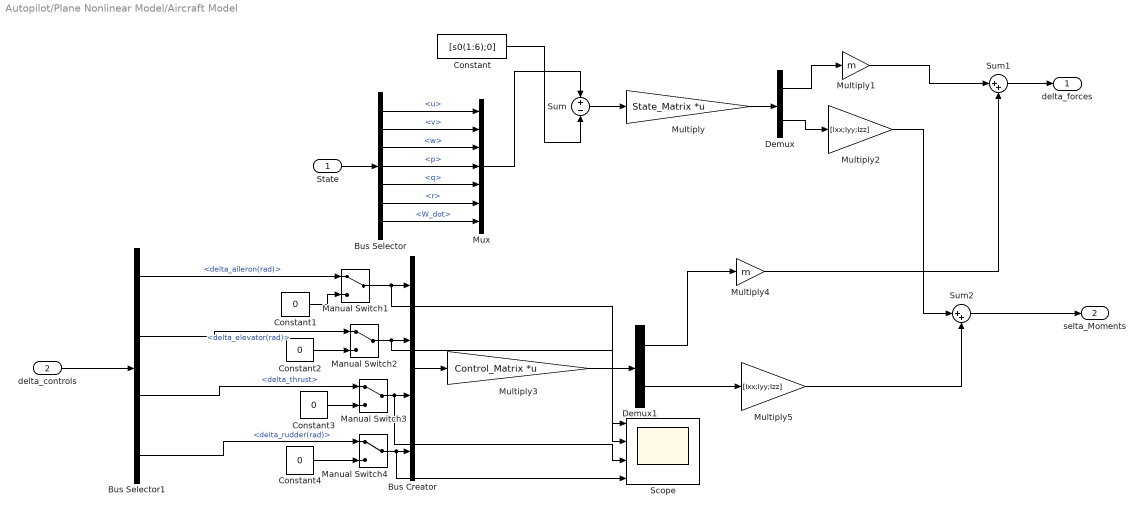
== system Autopilot/Plane Nonlinear Model/Aircraft Model ==
  State : Inport
  delta_controls : Inport  Port=2
  Bus Creator : BusCreator  Inputs=4
  Bus Selector : BusSelector  OutputSignals=u,v,w,p,q,r,W_dot
  Bus Selector1 : BusSelector  OutputSignals=Latr_control_actions.delta_aileron(rad),long_control_actions.delta_elevator(rad),long_control_actions.delta_thrust,Latr_control_actions.delta_rudder(rad)
  Constant : Constant  Value=[s0(1:6);0]
  Constant{1..4} (4 alike) : Constant  Value=0
  Demux : Demux  Outputs=2
  Demux1 : Demux  Outputs=2
  Manual Switch{1..4} (4 alike) : ManualSwitch
  Multiply : Gain  Gain=State_Matrix  Multiplication=Matrix(K*u) (u vector)
  Multiply1 : Gain  Gain=m
  Multiply2 : Gain  Gain=[Ixx;Iyy;Izz]
  Multiply3 : Gain  Gain=Control_Matrix  Multiplication=Matrix(K*u) (u vector)
  Multiply4 : Gain  Gain=m
  Multiply5 : Gain  Gain=[Ixx;Iyy;Izz]
  Mux : Mux  Inputs=7
  Scope : Scope  NumInputPorts=4
  Sum : Sum  Inputs=+-
  Sum1 : Sum  Inputs=|++
  Sum2 : Sum  Inputs=|++
  delta_forces : Outport
  selta_Moments : Outport  Port=2
  wires:
  State/1 -> Bus Selector/1
  Bus Selector/1 -> Mux/1  "<u>"
  Bus Selector/2 -> Mux/2  "<v>"
  Bus Selector/3 -> Mux/3  "<w>"
  Bus Selector/4 -> Mux/4  "<p>"
  Bus Selector/5 -> Mux/5  "<q>"
  Bus Selector/6 -> Mux/6  "<r>"
  Mux/1 -> Sum/1
  Constant/1 -> Sum/2
  Sum/1 -> Multiply/1
  Multiply/1 -> Demux/1
  Bus Selector/7 -> Mux/7  "<W_dot>"
  Demux/1 -> Multiply1/1
  Demux/2 -> Multiply2/1
  delta_controls/1 -> Bus Selector1/1
  Multiply3/1 -> Demux1/1
  Demux1/1 -> Multiply4/1
  Demux1/2 -> Multiply5/1
  Multiply4/1 -> Sum1/2
  Multiply1/1 -> Sum1/1
  Sum1/1 -> delta_forces/1
  Multiply2/1 -> Sum2/1
  Multiply5/1 -> Sum2/2
  Sum2/1 -> selta_Moments/1
  Bus Creator/1 -> Multiply3/1
  Manual Switch4/1 -> Scope/4, Bus Creator/4
  Manual Switch3/1 -> Scope/3, Bus Creator/3
  Manual Switch2/1 -> Scope/2, Bus Creator/2
  Manual Switch1/1 -> Scope/1, Bus Creator/1
  Constant1/1 -> Manual Switch1/2
  Constant2/1 -> Manual Switch2/2
  Constant3/1 -> Manual Switch3/2
  Constant4/1 -> Manual Switch4/2
  Bus Selector1/1 -> Manual Switch1/1  "<delta_aileron(rad)>"
  Bus Selector1/2 -> Manual Switch2/1  "<delta_elevator(rad)>"
  Bus Selector1/3 -> Manual Switch3/1  "<delta_thrust>"
  Bus Selector1/4 -> Manual Switch4/1  "<delta_rudder(rad)>"

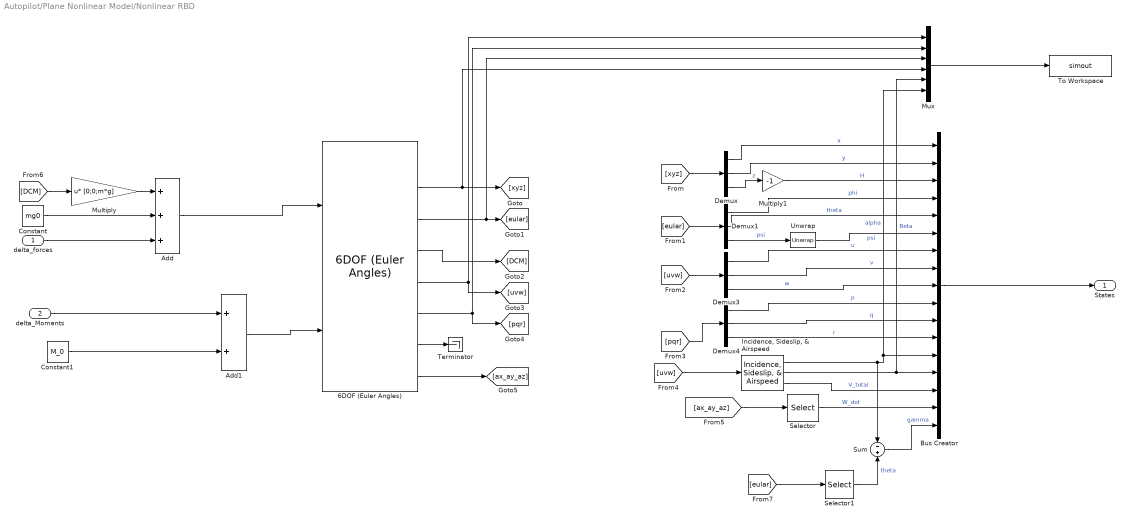
== system Autopilot/Plane Nonlinear Model/Nonlinear RBD ==
  delta_forces : Inport
  delta_Moments : Inport  Port=2
  6DOF (Euler Angles) : shared6dof/6DOF (Euler Angles)  units=English (Velocity in ft/s)  mtype=Fixed  rep=Euler Angles  xme_0=s0(10:12)  Vm_0=s0(1:3)  eul_0=s0(7:9)  pm_0=s0(4:6)  mass_0=m  mass_e=0.5  mass_f=2.0  inertia=I  inertia_e=eye(3)  inertia_f=2*eye(3)  k_quat=1.0  vre_flag=on  abi_flag=off  aMode=0  xme_statename=''  Vm_statename=''  eul_statename=''  quat_statename=''  pm_statename=''  mass_statename=''
  Add : Sum  Inputs=+++
  Add1 : Sum
  Bus Creator : BusCreator  Inputs=17
  Constant : Constant  Value=mg0
  Constant1 : Constant  Value=M_0
  Demux{,1,3..4} (4 alike) : Demux  Outputs=3
  "Incidence, Sideslip, & Airspeed" : aerolibasang/Incidence, Sideslip, & Airspeed
  Multiply : Gain  Gain=[0;0;m*g]  Multiplication=Matrix(u*K)
  Multiply1 : Gain  Gain=-1
  Mux : Mux  Inputs=6
  Selector : Selector  InputPortWidth=3  IndexOptions=Index vector (dialog)  Indices=3  OutputSizes=1
  Selector1 : Selector  InputPortWidth=3  IndexOptions=Index vector (dialog)  Indices=[2]  OutputSizes=1
  Sum : Sum  Inputs=-+
  Terminator : Terminator
  To Workspace : ToWorkspace  VariableName=simout  SaveFormat=Timeseries  SampleTime=-1
  Unwrap : dspsigops/Unwrap  tol=pi  InputProcessing=Columns as channels (frame based)  running=off
  States : Outport
  wires:
  6DOF (Euler Angles)/4 -> [DCM]
  Demux1/2 -> Bus Creator/5  "theta"
  6DOF (Euler Angles)/2 -> [xyz], Mux/4
  "Incidence, Sideslip, & Airspeed"/2 -> Bus Creator/14, Mux/5  "Beta"
  Demux/3 -> Multiply1/1  "z"
  Demux3/2 -> Bus Creator/8  "v"
  Constant/1 -> Add/2
  Add/1 -> 6DOF (Euler Angles)/1
  delta_Moments/1 -> Add1/1
  Demux/2 -> Bus Creator/2  "y"
  Demux1/3 -> Unwrap/1  "psi"
  Demux3/3 -> Bus Creator/9  "w"
  6DOF (Euler Angles)/6 -> [pqr], Mux/2
  [DCM] -> Multiply/1
  [uvw] -> Demux3/1
  6DOF (Euler Angles)/3 -> [eular], Mux/3
  [xyz] -> Demux/1
  [pqr] -> Demux4/1
  Demux1/1 -> Bus Creator/4  "phi"
  Demux4/2 -> Bus Creator/11  "q"
  Demux3/1 -> Bus Creator/7  "u"
  Demux/1 -> Bus Creator/1  "x"
  delta_forces/1 -> Add/3
  Demux4/3 -> Bus Creator/12  "r"
  Demux4/1 -> Bus Creator/10  "p"
  Multiply/1 -> Add/1
  Selector/1 -> Bus Creator/16  "W_dot"
  "Incidence, Sideslip, & Airspeed"/1 -> Sum/1, Mux/6, Bus Creator/13  "alpha"
  "Incidence, Sideslip, & Airspeed"/3 -> Bus Creator/15  "V_total"
  [uvw] -> "Incidence, Sideslip, & Airspeed"/1
  [ax_ay_az] -> Selector/1
  Constant1/1 -> Add1/2
  Add1/1 -> 6DOF (Euler Angles)/2
  Bus Creator/1 -> States/1
  6DOF (Euler Angles)/5 -> [uvw], Mux/1
  Mux/1 -> To Workspace/1
  6DOF (Euler Angles)/8 -> [ax_ay_az]
  Multiply1/1 -> Bus Creator/3  "H"
  Sum/1 -> Bus Creator/17  "gamma"
  Selector1/1 -> Sum/2  "theta"
  6DOF (Euler Angles)/7 -> Terminator/1
  [eular] -> Selector1/1
  [eular] -> Demux1/1
  Unwrap/1 -> Bus Creator/6  "psi"

== system Autopilot/Subsystem/Gamma & H ==
  u : Inport
  w : Inport  Port=2
  theta : Inport  Port=3
  Atan2 : Trigonometry  Operator=atan2
  Constant12 : Constant  Value=-z_0
  Gain3 : Gain  Gain=R2D
  Hypot : Math  Operator=hypot
  Integrator : Integrator
  Product : Product
  Sin : Trigonometry
  Sum3 : Sum  Inputs=|+-
  Sum4 : Sum  Inputs=|++
  H : Outport
  gamma_deg : Outport  Port=2
  tag scope: HH=global
  wires:
  u/1 -> Hypot/1, Atan2/2
  Sum3/1 -> Gain3/1, Sin/1  "gamma"
  w/1 -> Hypot/2, Atan2/1
  Integrator/1 -> Sum4/1
  Product/1 -> Integrator/1  "delta _hdot"
  Sin/1 -> Product/2
  Atan2/1 -> Sum3/2  "Alpha"
  Constant12/1 -> Sum4/2
  Hypot/1 -> Product/1  "v_tot"
  theta/1 -> Sum3/1
  Gain3/1 -> gamma_deg/1
  Sum4/1 -> [HH], H/1

== matlab function Autopilot/Subsystem/MATLAB Function ==
  data: u_v_w input; Xe_dot output; phi_theta_psi input; Ye_dot output; Ze_dot output
function [Xe_dot, Ye_dot, Ze_dot] = fcn(u_v_w, phi_theta_psi)
    u = u_v_w(1);
    v = u_v_w(2);
    w = u_v_w(3);
    phi = phi_theta_psi(1);
    theta = phi_theta_psi(2);
    psi = phi_theta_psi(3);

    T = [
        cos(theta)*cos(psi), sin(phi)*sin(theta)*cos(psi) - cos(phi)*sin(psi), cos(phi)*sin(theta)*cos(psi) + sin(phi)*sin(psi);
        cos(theta)*sin(psi), sin(phi)*sin(theta)*sin(psi) + cos(phi)*cos(psi), cos(phi)*sin(theta)*sin(psi) - sin(phi)*cos(psi);
        -sin(theta),          sin(phi)*cos(theta),                           cos(phi)*cos(theta)
    ];

    XYZ_E_dot = T * [u; v; w];
    Xe_dot = XYZ_E_dot(1);
    Ye_dot = XYZ_E_dot(2);
    Ze_dot = XYZ_E_dot(3);
end
